simulink model "pendulo"  (R2020b)
settings: Solver=VariableStepAuto  StartTime=0.0  StopTime=100  RelTol=1e-3
values from neighbouring files (symbols this model uses):
  controlador = projetarControlador(requisitos, planta)    [executarTudo.m]    (also in runAll.m; simular.m)
  planta = obterPlanta()    [codetest.m]    (also in executarTudo.m; nextState.m; runAll.m; simular.m)
  thetar = 0    [executarTudo.m]    (also in runAll.m)
undefined symbols (not defined in the file or in its folder): varCom, varMed
libraries: pid_lib x1
settings Model: Creator=davi  LastModifiedBy=alexandremaranhao

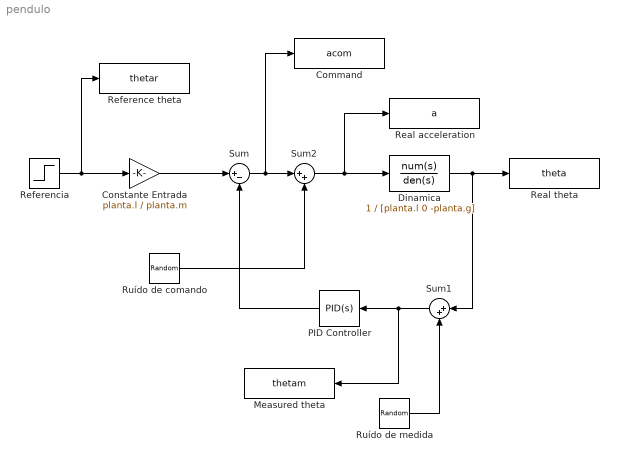
== system pendulo ==
  Command : ToWorkspace  VariableName=acom  SaveFormat=Structure With Time  SampleTime=-1
  Constante Entrada : Gain  Gain=planta.l / planta.m
  Dinamica : TransferFcn  Numerator=1  Denominator=[planta.l 0 -planta.g]
  Measured theta : ToWorkspace  VariableName=thetam  SaveFormat=Structure With Time  SampleTime=-1
  PID Controller : pid_lib/PID Controller  Controller=PID  Form=Parallel  TimeDomain=Continuous-time  UseExternalTs=off  SampleTime=-1  IntegratorMethod=Forward Euler  FilterMethod=Forward Euler  ControllerParametersSource=internal  P=controlador.Kp  I=0  D=controlador.Kd  UseFilter=on  N=100  TunerSelectOption=Transfer Function Based (PID Tuner App)  InitialConditionSource=internal  InitialConditionForIntegrator=0  InitialConditionForFilter=0  DifferentiatorICPrevScaledInput=0  ExternalReset=none  TrackingMode=off  Kt=1  LimitOutput=off  SatLimitsSource=internal  UpperSaturationLimit=inf  LowerSaturationLimit=-inf  LinearizeAsGain=on  AntiWindupMode=none  Kb=1  POutMin=[]  POutMax=[]  IOutMin=[]  IOutMax=[]  DOutMin=[]  DOutMax=[]  NOutMin=[]  NOutMax=[]  SumOutMin=[]  SumOutMax=[]  SaturationOutMin=[]  SaturationOutMax=[]  PParamMin=[]  PParamMax=[]  IParamMin=[]  IParamMax=[]  DParamMin=[]  DParamMax=[]  NParamMin=[]  NParamMax=[]  KbParamMin=[]  KbParamMax=[]  KtParamMin=[]  KtParamMax=[]  KbOutMin=[]  KbOutMax=[]  KtOutMin=[]  KtOutMax=[]  IntegratorOutMin=[]  IntegratorOutMax=[]  FilterOutMin=[]  FilterOutMax=[]  SumI1OutMin=[]  SumI1OutMax=[]  SumI2OutMin=[]  SumI2OutMax=[]  SumI3OutMin=[]  SumI3OutMax=[]  SumI4OutMin=[]  SumI4OutMax=[]  SumDOutMin=[]  SumDOutMax=[]  DifferentiatorOutMin=[]  DifferentiatorOutMax=[]  FilterDiffOutCoefMin=[]  FilterDiffOutCoefMax=[]  ReciprocalOutMin=[]  ReciprocalOutMax=[]  SumDenOutMin=[]  SumDenOutMax=[]  SumNumOutMin=[]  SumNumOutMax=[]  DivideOutMin=[]  DivideOutMax=[]  UdiffTsProdOutMin=[]  UdiffTsProdOutMax=[]  NTsProdOutMin=[]  NTsProdOutMax=[]  UintegralTsProdOutMin=[]  UintegralTsProdOutMax=[]  UngainTsProdOutMin=[]  UngainTsProdOutMax=[]  IntegratorContinuousStateAttributes=''  IntegratorStateMustResolveToSignalObject=off  IntegratorRTWStateStorageClass=Auto  FilterContinuousStateAttributes=''  FilterStateMustResolveToSignalObject=off  FilterRTWStateStorageClass=Auto  ParallelPVariant=InternalParameters  IdealPVariant=Disabled  IVariant=InternalParameters  DVariant=InternalParameters  IntegratorVariant=Continuous  SatVariant=Disabled  AWVariant=Passthrough  PCopyVariant=Disabled  TRVariant=Disabled  FdbkBlocksVariant=Forward  IdealPFdbkVariant=Disabled  SatFdbkVariant=Disabled  DerivativeFilterVariant=ContFilter  NVariant=InternalParameters  NCopyVariant=Disabled  FilterICVariant=InternalICsFilter  IntegratorICVariant=InternalICs  ExternalResetVariant=Disabled  TRSumVariant=Passthrough  SumFdbkVariant=Disabled  SumVariant=Sum_PID  TsampFilterVariant=InternalTs  TsampNgainVariant=Passthrough  TsampIntegralVariant=Passthrough  ExternalSaturationOutDataTypeStr=Inherit: Same as second input
  Real acceleration : ToWorkspace  VariableName=a  SaveFormat=Structure With Time  SampleTime=-1
  Real theta : ToWorkspace  VariableName=theta  SaveFormat=Structure With Time  SampleTime=-1
  Reference theta : ToWorkspace  VariableName=thetar  SaveFormat=Structure With Time  SampleTime=-1
  Referencia : Step  Time=0  After=thetar  SampleTime=0
  Ruído de comando : RandomNumber  Variance=varCom  SampleTime=0.1
  Ruído de medida : RandomNumber  Variance=varMed  SampleTime=0.1
  Sum : Sum  Inputs=|+-
  Sum1 : Sum  Inputs=|++
  Sum2 : Sum  Inputs=|++
  wires:
  Referencia/1 -> Reference theta/1, Constante Entrada/1
  Constante Entrada/1 -> Sum/1
  Dinamica/1 -> Sum1/1, Real theta/1
  PID Controller/1 -> Sum/2
  Sum/1 -> Sum2/1, Command/1
  Ruído de medida/1 -> Sum1/2
  Sum1/1 -> Measured theta/1, PID Controller/1
  Sum2/1 -> Real acceleration/1, Dinamica/1
  Ruído de comando/1 -> Sum2/2
